simulink model "sample01"  (R2018b)
settings: Solver=VariableStepAuto  StartTime=0.0  StopTime=100  RelTol=1e-3
libraries: simulink x1
settings Model: Creator=chpark  LastModifiedBy=chpark

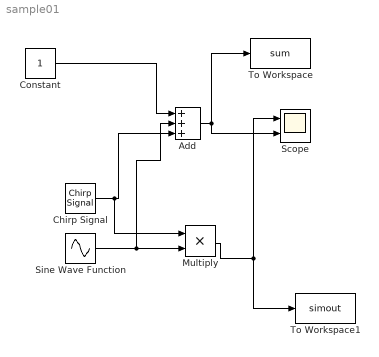
== system sample01 ==
  Add : Sum  Inputs=+++
  Chirp Signal : simulink/Sources/Chirp Signal  f1=0.1  T=100  f2=1
  Constant : Constant
  Multiply : Product
  Scope : Scope  NumInputPorts=2
  Sine Wave Function : Sin  TimeSource=Use external signal  SampleTime=0
  To Workspace : ToWorkspace  VariableName=sum  SaveFormat=Timeseries  SampleTime=-1
  To Workspace1 : ToWorkspace  VariableName=simout  SaveFormat=Timeseries  SampleTime=-1
  wires:
  Constant/1 -> Add/1
  Chirp Signal/1 -> Multiply/1, Add/3
  Sine Wave Function/1 -> Add/2, Multiply/2
  Add/1 -> To Workspace/1, Scope/2
  Multiply/1 -> Scope/1, To Workspace1/1
